simulink model "ejxtmn"  (Simulink 5.0)
settings: Solver=ode45  StartTime=0.0  StopTime=10.0  RelTol=1e-3
settings Model: LastModifiedBy=强鹏俊

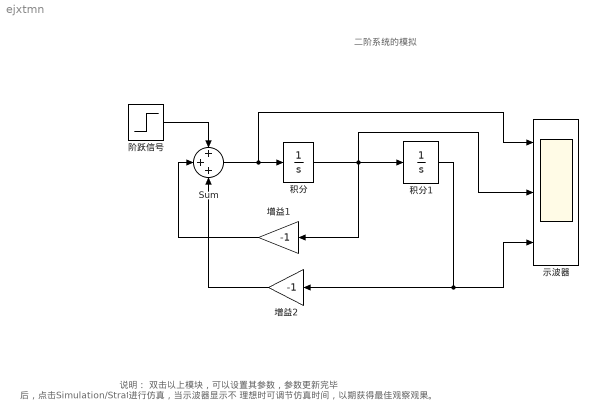
== system ejxtmn ==
  note: 二阶系统的模拟
  note: 说明：
      |        双击以上模块，可以设置其参数，参数更新完毕
      | 后，点击Simulation/Strat进行仿真，当示波器显示不
      | 理想时可调节仿真时间，以期获得最佳观察观果。
  Sum : Sum  Inputs=+++  SaturateOnIntegerOverflow=on
  积分 : Integrator
  积分1 : Integrator
  阶跃信号 : Step  SampleTime=0
  示波器 : Scope  NumInputPorts=3
      settings: TimeRange=10  YMin=-5~-5~-5  YMax=5~5~5
  增益1 : Gain  Orientation=left  Gain=-1  SaturateOnIntegerOverflow=on
  增益2 : Gain  Orientation=left  Gain=-1  SaturateOnIntegerOverflow=on
  wires:
  阶跃信号/1 -> Sum/1
  Sum/1 -> 积分/1, 示波器/1
  增益1/1 -> Sum/2
  积分1/1 -> 增益2/1, 示波器/3
  增益2/1 -> Sum/3
  积分/1 -> 增益1/1, 积分1/1, 示波器/2
